simulink model "EngTrqPtd_CoOfs"  (R2016b)
settings: configuration reference "CodeGenConfigSet" (kept outside this file)
values from neighbouring files (symbols this model uses):
  EngTrqPtd_stPthLim_C = Calibration.Parameter    [init_EngTrqPtd_CoOfs.m]
  EngTrqPtd_trqLim_C = Calibration.Parameter    [init_EngTrqPtd_CoOfs.m]
settings Model: Creator=Wollf  LastModifiedBy=Wollf
settings ConfigSetRef: SourceLocation=Base Workspace

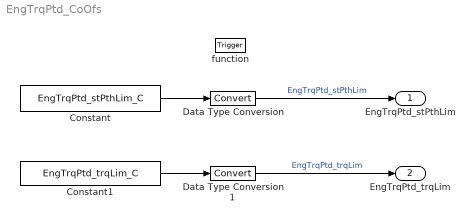
== system EngTrqPtd_CoOfs ==
  function : TriggerPort  TriggerType=function-call  VariantControl=Variant
  Constant : Constant  Value=EngTrqPtd_stPthLim_C
  Constant1 : Constant  Value=EngTrqPtd_trqLim_C
  Data Type Conversion : DataTypeConversion
  Data Type Conversion1 : DataTypeConversion
  EngTrqPtd_stPthLim : Outport  Description=State of engine torque limitation from ECU monitoring  OutMin=0  OutMax=255  OutDataTypeStr=State_uint8
  EngTrqPtd_trqLim : Outport  Tag=Nm  Description=Set path torque limitation from ECU monitoring  Port=2  OutMin=-3276  OutMax=3276  OutDataTypeStr=Trq_Nm
  wires:
  Constant/1 -> Data Type Conversion/1
  Constant1/1 -> Data Type Conversion1/1
  Data Type Conversion/1 -> EngTrqPtd_stPthLim/1  "EngTrqPtd_stPthLim"
  Data Type Conversion1/1 -> EngTrqPtd_trqLim/1  "EngTrqPtd_trqLim"
